simulink model "bldc_pid_2016"  (R2022b)
settings: Solver=FixedStepAuto  StartTime=0.0  StopTime=t_max  FixedStep=1/1000  RelTol=1e-3
values from neighbouring files (symbols this model uses):
  D = 1e-4    (= 0.0001)    [script.m]
  J = 1e-5    (= 1e-05)    [script.m]
  Kb = 0.1433    [script.m]
  Kt = 0.1433    [script.m]
  L = 0.052    [script.m]
  R = 21.2    [script.m]
  step_v = 1000    [script.m]
undefined symbols (not defined in the file or in its folder): Kp, Td, Ti
settings Model: Creator=ricar  LastModifiedBy=mluser
settings SolverCC: AlgebraicLoopSolver=TrustRegion
settings DataIOCC: ReturnWorkspaceOutputs=off
settings DebuggingCC: UnconnectedInputMsg=warning  UnconnectedOutputMsg=warning  UnconnectedLineMsg=warning  SFMachineParentedDataDiag=warning  ArithmeticOperatorsInVariantConditions=warning
settings ModelReferenceCC: EnableRefExpFcnMdlSchedulingChecks=on
settings SFSimCC: SimUseLocalCustomCode=off  CustomCodeUndefinedFunction=UseInterfaceOnly
settings RTWCC: RTWUseLocalCustomCode=off
settings CodeAppCC: StateflowObjectComments=on

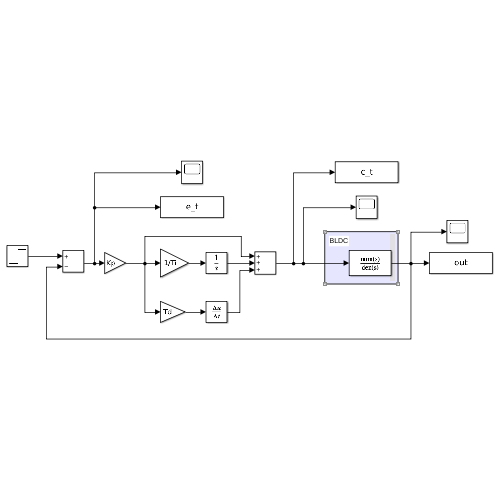
[thumbnail: Simulink's stored preview of the top-level diagram]
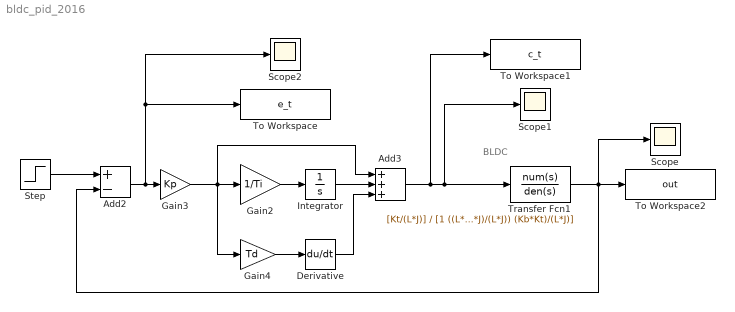
== system bldc_pid_2016 ==
  note: BLDC
  Add2 : Sum  Inputs=+-
  Add3 : Sum  Inputs=+++
  Derivative : Derivative
  Gain2 : Gain  Gain=1/Ti
  Gain3 : Gain  Gain=Kp
  Gain4 : Gain  Gain=Td
  Integrator : Integrator
  Scope : Scope
  Scope1 : Scope
  Scope2 : Scope
  Step : Step  Time=0  After=step_v  SampleTime=0
  To Workspace : ToWorkspace  VariableName=e_t  SampleTime=-1
  To Workspace1 : ToWorkspace  VariableName=c_t  SampleTime=-1
  To Workspace2 : ToWorkspace  VariableName=out  SampleTime=-1
  Transfer Fcn1 : TransferFcn  Numerator=[Kt/(L*J)]  Denominator=[1 ((L*D+R*J)/(L*J)) (Kb*Kt)/(L*J)]
  wires:
  Transfer Fcn1/1 -> To Workspace2/1, Scope/1, Add2/2
  Step/1 -> Add2/1
  Gain2/1 -> Integrator/1
  Gain4/1 -> Derivative/1
  Add2/1 -> Gain3/1, Scope2/1, To Workspace/1
  Integrator/1 -> Add3/2
  Derivative/1 -> Add3/3
  Add3/1 -> To Workspace1/1, Transfer Fcn1/1, Scope1/1
  Gain3/1 -> Gain2/1, Gain4/1, Add3/1
